simulink model "SMC_simulink"  (R2018a)
settings: Solver=FixedStepAuto  StartTime=0.0  StopTime=3000  FixedStep=1e-2  RelTol=1e-3
settings Model: PacingRate=100  Creator=MinhKhanhPC  LastModifiedBy=thanhdo
settings SolverCC: ZeroCrossAlgorithm=Adaptive
settings DebuggingCC: MaxConsecutiveZCsMsg=none

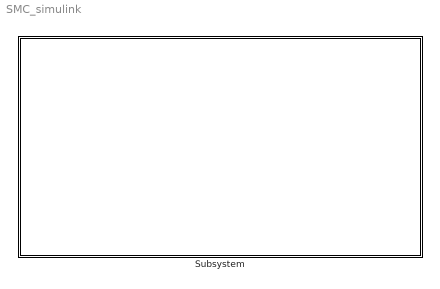
== system SMC_simulink ==
  Subsystem : Subsystem  mask{upper_limit=[2.28e-5 4.28e-5]}

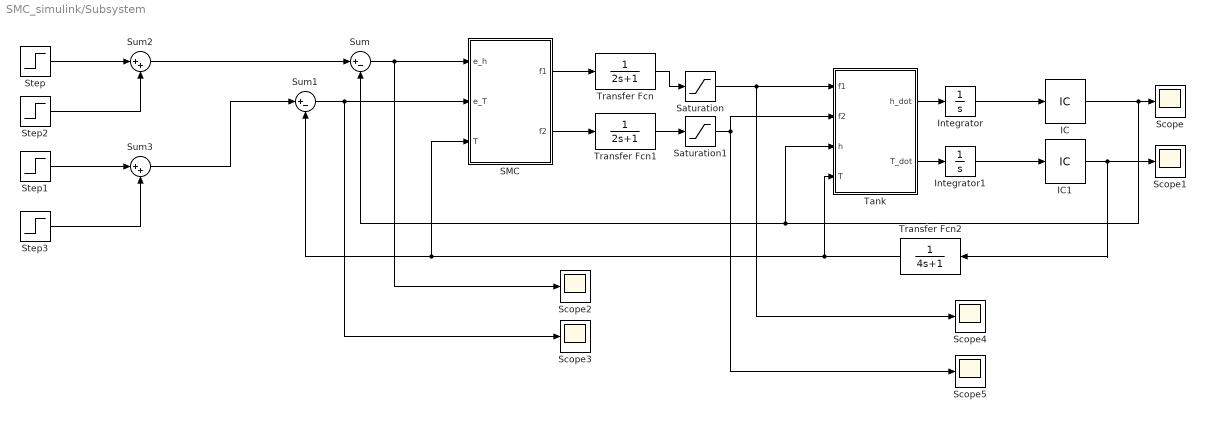
== system SMC_simulink/Subsystem ==
  IC : InitialCondition  Value=0.18
  IC1 : InitialCondition  Value=35
  Integrator : Integrator  InitialCondition=0.18
  Integrator1 : Integrator  InitialCondition=35
  SMC : MATLAB Function  TreatAsAtomicUnit=on
  Saturation : Saturate  UpperLimit=upper_limit(1)  LowerLimit=0
  Saturation1 : Saturate  UpperLimit=upper_limit(2)  LowerLimit=0
  Scope{,1..5} (6 alike) : Scope
  Step : Step  After=0.2  SampleTime=0
  Step1 : Step  After=40  SampleTime=0
  Step2 : Step  Time=400  After=-0.05  SampleTime=0
  Step3 : Step  Time=600  After=10  SampleTime=0
  Sum : Sum  Inputs=|+-
  Sum1 : Sum  Inputs=|+-
  Sum2 : Sum  Inputs=|++
  Sum3 : Sum  Inputs=|++
  Tank : MATLAB Function  TreatAsAtomicUnit=on
  Transfer Fcn : TransferFcn  Denominator=[2 1]
  Transfer Fcn1 : TransferFcn  Denominator=[2 1]
  Transfer Fcn2 : TransferFcn  Denominator=[4 1]
  wires:
  IC/1 -> Tank/3(h), Sum/2, Scope/1
  Tank/1(h_dot) -> Integrator/1
  Integrator/1 -> IC/1
  Integrator1/1 -> IC1/1
  SMC/2(f2) -> Transfer Fcn1/1
  Tank/2(T_dot) -> Integrator1/1
  Sum1/1 -> Scope3/1, SMC/2(e_T)
  Sum/1 -> Scope2/1, SMC/1(e_h)
  IC1/1 -> Scope1/1, Transfer Fcn2/1
  Step/1 -> Sum2/1
  Step2/1 -> Sum2/2
  Sum2/1 -> Sum/1
  Step1/1 -> Sum3/1
  Step3/1 -> Sum3/2
  Sum3/1 -> Sum1/1
  Transfer Fcn/1 -> Saturation/1
  Transfer Fcn1/1 -> Saturation1/1
  Saturation/1 -> Scope4/1, Tank/1(f1)
  SMC/1(f1) -> Transfer Fcn/1
  Saturation1/1 -> Tank/2(f2), Scope5/1
  Transfer Fcn2/1 -> Tank/4(T), SMC/3(T), Sum1/2

== matlab function SMC_simulink/Subsystem/SMC ==
  settings: updateMethod=DISCRETE
  data: e_h input; e_T input; f1 output; T input; f2 output
function [f1,f2]  = fcn(e_h,e_T,T)
%e=[e1 e2]=[e_h e_T]
%f= [f1 f2]= [f_cold f_hot]
%y= [h T]
A=3.24e-2; % tank cross area
T_hot=70; % hot temperature
T_cold=20; % cold temperature

g=9.81; % gravity coefficient
%a0=pi*(0.021/2)^2; % pipe cross erea

%v=0.5; % valve open

%alpha=sqrt(2*g)*v*a0; % f_valve= alpha*sqrt(h)
%upper_limit=3e-4;


k_1=35;
k_2=0.2;
% f3= alpha*sqrt(h); % or use alpha*sqrt(h)

%%f3_max=alpha*sqrt(0.3);
f3_max=4.7e-5;

% f1= A*(k_1*sign(e_T)-(k+f3_max)*sign(e_h)*(T_hot-T))/(T_cold-T_hot);

% f2= A*(k_1*sign(e_T)-(k+f3_max)*sign(e_h)*(T_cold-T))/(T_hot-T_cold);

f1= A*(k_2*tanh(e_T)-(k_1+f3_max)*tanh(e_h)*(T_hot-T))/(T_cold-T_hot);

f2= A*(k_2*tanh(e_T)-(k_1+f3_max)*tanh(e_h)*(T_cold-T))/(T_hot-T_cold);

% if h>0.3
%     f1=0;
%     f2=0;
% end

== matlab function SMC_simulink/Subsystem/Tank ==
  settings: updateMethod=DISCRETE
  data: f1 input; h_dot output; f2 input; T_dot output; h input; T input
function [h_dot,T_dot]  = fcn(f1,f2,h,T)
%y=[h, T]
%y_dot= [h_dot, T_dot]
A=3.24e-2;
T_hot=70;
T_cold=20;

%g=9.81;
%a0=pi*(0.021/2)^2;

%v=0.5;

%a=v*a0;


%alpha=sqrt(2*g)*a;
%f3=alpha*sqrt(h); 
f3=4.7e-5/sqrt(0.3)*sqrt(h);

h_dot=(f1+f2-f3)/A;
T_dot=(f1.*(T_cold-T)+f2.*(T_hot- T))/(A*h);
